simulink model "Electrical"  (R2022b)
settings: Solver=VariableStepAuto  StartTime=0.0  StopTime=10.0  RelTol=1e-3
model workspace (MAT data in the model file):
  QL = Simulink.Parameter
  QL.Value = 960000
  QL.DataType = 'auto'
  QL.Complexity = 'real'
  QL.Dimensions = [1 1]
  RL = Simulink.Parameter
  RL.Value = Simulink.data.Expression
  RL.Value.ExpressionString = "QL*RQ"
  RL.DataType = 'auto'
  RL.Complexity = 'real'
  RL.Dimensions = -1
  RQ = Simulink.Parameter
  RQ.Value = 310
  RQ.DataType = 'auto'
  RQ.Complexity = 'real'
  RQ.Dimensions = [1 1]
  Ts = Simulink.Parameter
  Ts.Value = 1e-10
  Ts.DataType = 'auto'
  Ts.Complexity = 'real'
  Ts.Dimensions = [1 1]
  f0 = Simulink.Parameter
  f0.Value = 648000000
  f0.DataType = 'auto'
  f0.Complexity = 'real'
  f0.Dimensions = [1 1]
  w_hbw = Simulink.Parameter
  w_hbw.Value = Simulink.data.Expression
  w_hbw.Value.ExpressionString = "2*pi*f0/QL"
  w_hbw.DataType = 'auto'
  w_hbw.Complexity = 'real'
  w_hbw.Dimensions = -1
settings Model: Creator=mliu  LastModifiedBy=mliu

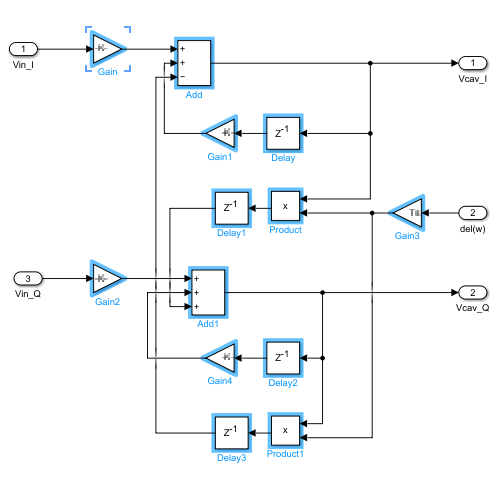
[thumbnail: Simulink's stored preview of the top-level diagram]
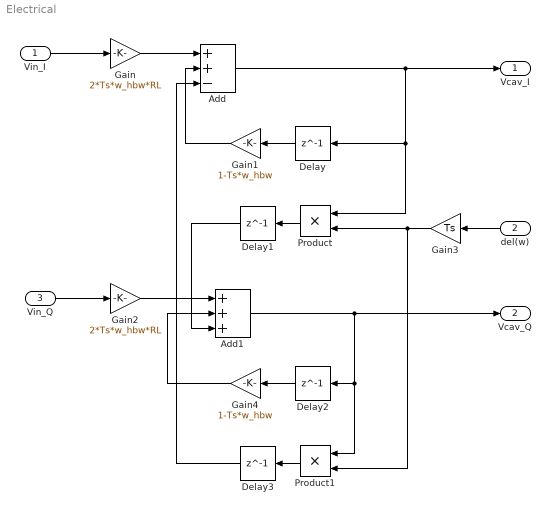
== system Electrical ==
  Vin_I : Inport
  del(w) : Inport  Port=2
  Vin_Q : Inport  Port=3
  Add : Sum  Inputs=++-
  Add1 : Sum  Inputs=+++
  Delay{,1..3} (4 alike) : Delay  DelayLength=1  InitialCondition=0
  Gain : Gain  Gain=2*Ts*w_hbw*RL
  Gain1 : Gain  Gain=1-Ts*w_hbw
  Gain2 : Gain  Gain=2*Ts*w_hbw*RL
  Gain3 : Gain  Gain=Ts
  Gain4 : Gain  Gain=1-Ts*w_hbw
  Product : Product
  Product1 : Product
  Vcav_I : Outport
  Vcav_Q : Outport  Port=2
  wires:
  Vin_I/1 -> Gain/1
  Gain/1 -> Add/1
  Add/1 -> Product/1, Delay/1, Vcav_I/1
  Delay/1 -> Gain1/1
  Gain1/1 -> Add/2
  Product/1 -> Delay1/1
  Vin_Q/1 -> Gain2/1
  Gain2/1 -> Add1/1
  Delay1/1 -> Add1/3
  Add1/1 -> Product1/1, Delay2/1, Vcav_Q/1
  del(w)/1 -> Gain3/1
  Gain3/1 -> Product1/2, Product/2
  Delay2/1 -> Gain4/1
  Gain4/1 -> Add1/2
  Product1/1 -> Delay3/1
  Delay3/1 -> Add/3
